simulink model "wetmodel_fixed_angle_r2020"  (R2020b)
settings: Solver=ode45  StartTime=0.0  StopTime=45  RelTol=1e-3  EnableMultiTasking=on
libraries: dspsigops x1
settings Model: Tag=MP_system  Creator=Andries  LastModifiedBy=jurre
settings DataIOCC: LimitDataPoints=on  SaveFormat=Array  SignalLoggingSaveFormat=ModelDataLogs  ReturnWorkspaceOutputs=off
settings OptimizationCC: ExpressionDepthLimit=2147483647  LifeSpan=inf
settings DebuggingCC: UnderspecifiedInitializationDetection=Classic  MergeDetectMultiDrivingBlocksExec=none  SolverPrmCheckMsg=warning  FcnCallInpInsideContextMsg=warning  StateNameClashWarn=warning  SFUnexpectedBacktrackingDiag=warning  SFNoUnconditionalDefaultTransitionDiag=warning  SFExecutionAtInitializationDiag=none  ArithmeticOperatorsInVariantConditions=warning
settings HardwareCC: ProdBitPerPointer=32  ProdBitPerSizeT=32  ProdBitPerPtrDiffT=32  ProdLargestAtomicFloat=None  ProdIntDivRoundTo=Undefined  ProdEndianess=Unspecified  ProdWordSize=32  ProdHWDeviceType=32-bit Generic
settings ModelReferenceCC: PropagateSignalLabelsOutOfModel=off
settings SFSimCC: SimUseLocalCustomCode=off  CustomCodeUndefinedFunction=UseInterfaceOnly
settings RTWCC: RTWUseLocalCustomCode=off
settings CodeAppCC: StateflowObjectComments=on
settings GRTTargetCC: TargetLangStandard=C89/C90 (ANSI)  CombineOutputUpdateFcns=off  GRTInterface=on
settings ConfigComp: CovMetricSettings=dw  CovSaveCumulativeToWorkspaceVar=on  CovSaveSingleToWorkspaceVar=on  CovExternalEMLEnable=off
settings SimscapeCC: SimscapeNormalizeSystem=off

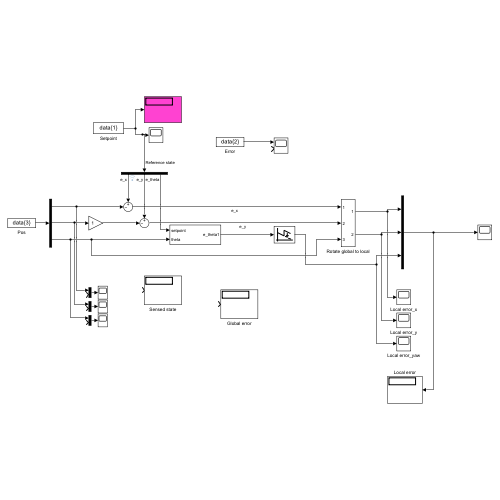
[thumbnail: Simulink's stored preview of the top-level diagram]
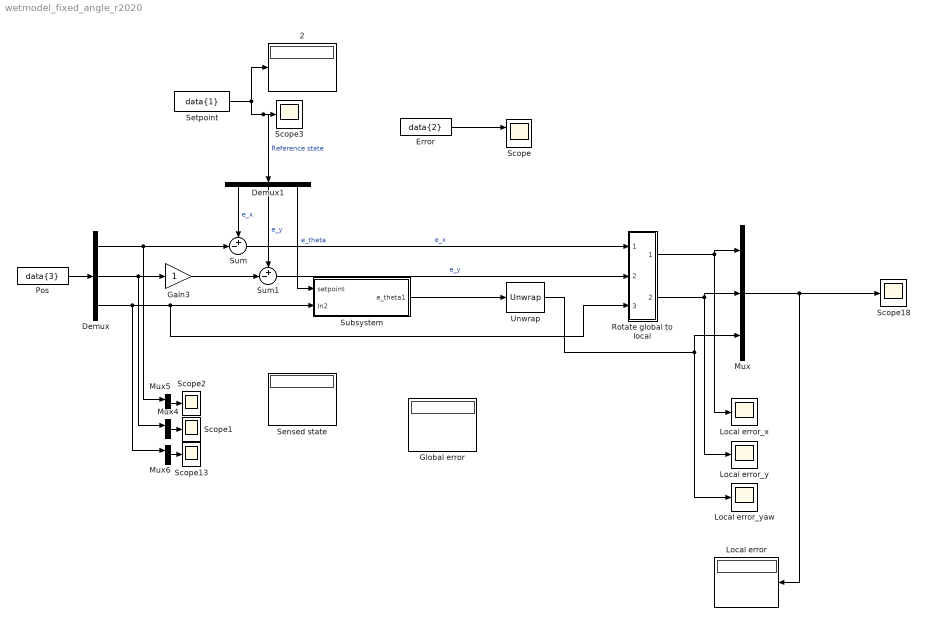
== system wetmodel_fixed_angle_r2020 ==
  "  2" : Display
  Demux : Demux  Outputs=3
  Demux1 : Demux  Outputs=3
  Error : FromWorkspace  VariableName=data{2}
  Gain3 : Gain
  Global error : Display
  Local error : Display
  "Local error_x " : Scope
  "Local error_y " : Scope
  "Local error_yaw " : Scope
  Mux : Mux  Inputs=3
  Mux4 : Mux  Inputs=2
  Mux5 : Mux  Inputs=2
  Mux6 : Mux  Inputs=2
  Pos : FromWorkspace  VariableName=data{3}
  "Rotate global to local " : Subsystem
  Scope : Scope  NumInputPorts=2
  Scope{1..3,13,18} (5 alike) : Scope
  Sensed state : Display
  Setpoint : FromWorkspace  VariableName=data{1}  OutputAfterFinalValue=Holding final value
  Subsystem : Subsystem
  Sum : Sum  Inputs=+-|
  Sum1 : Sum  Inputs=+-|
  Unwrap : dspsigops/Unwrap  tol=pi  InputProcessing=Columns as channels (frame based)  running=off
  wires:
  Setpoint/1 -> "  2"/1, Demux1/1, Scope3/1  "Reference state"
  Sum1/1 -> "Rotate global to local "/2(In2)  "e_y"
  Sum/1 -> "Rotate global to local "/1(In1)  "e_x"
  Mux/1 -> Local error/1, Scope18/1
  "Rotate global to local "/1(Out1) -> Mux/1, "Local error_x "/1
  Demux/1 -> Sum/2, Mux5/1
  Demux/2 -> Mux4/1, Gain3/1
  Demux/3 -> "Rotate global to local "/3(In3), Subsystem/2(In2), Mux6/1
  "Rotate global to local "/2(Out2) -> Mux/2, "Local error_y "/1
  Unwrap/1 -> Mux/3, "Local error_yaw "/1
  Mux6/1 -> Scope13/1
  Mux4/1 -> Scope1/1
  Mux5/1 -> Scope2/1
  Gain3/1 -> Sum1/2
  Pos/1 -> Demux/1
  Error/1 -> Scope/1
  Demux1/1 -> Sum/1  "e_x"
  Demux1/2 -> Sum1/1  "e_y"
  Demux1/3 -> Subsystem/1(setpoint)  "e_theta"
  Subsystem/1(e_theta1) -> Unwrap/1

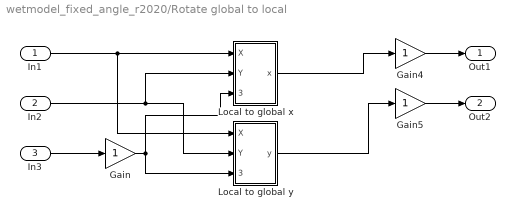
== system wetmodel_fixed_angle_r2020/Rotate global to local  ==
  In1 : Inport
  In2 : Inport  Port=2
  In3 : Inport  Port=3
  Gain : Gain
  Gain4 : Gain
  Gain5 : Gain
  "Local to global x " : Subsystem
  Local to global y : Subsystem
  Out1 : Outport  VectorParamsAs1DForOutWhenUnconnected=off
  Out2 : Outport  Port=2  VectorParamsAs1DForOutWhenUnconnected=off
  wires:
  Local to global y/1(y) -> Gain5/1
  In2/1 -> Local to global y/2(Y), "Local to global x "/2(Y)
  "Local to global x "/1(x) -> Gain4/1
  In1/1 -> Local to global y/1(X), "Local to global x "/1(X)
  In3/1 -> Gain/1
  Gain/1 -> Local to global y/3(theta), "Local to global x "/3(theta)
  Gain5/1 -> Out2/1
  Gain4/1 -> Out1/1

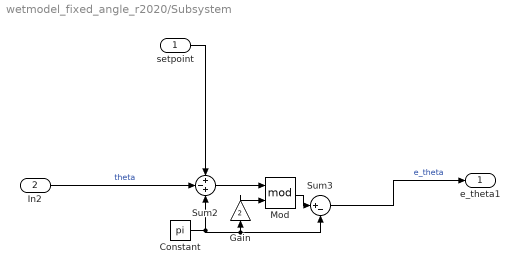
== system wetmodel_fixed_angle_r2020/Subsystem ==
  setpoint : Inport
  In2 : Inport  Port=2
  Constant : Constant  Value=pi
  Gain : Gain  Gain=2
  Mod : Math  Operator=mod  SaturateOnIntegerOverflow=on
  Sum2 : Sum  Inputs=+-+
  Sum3 : Sum  Inputs=|+-
  e_theta1 : Outport
  wires:
  setpoint/1 -> Sum2/1
  Mod/1 -> Sum3/1
  Constant/1 -> Sum3/2, Gain/1, Sum2/3
  In2/1 -> Sum2/2  "theta"
  Gain/1 -> Mod/2
  Sum2/1 -> Mod/1
  Sum3/1 -> e_theta1/1  "e_theta"

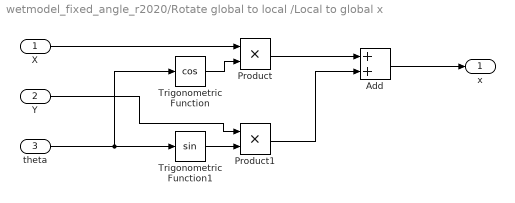
== system wetmodel_fixed_angle_r2020/Rotate global to local /Local to global x  ==
  X : Inport
  Y : Inport  Port=2
  theta : Inport  Port=3
  Add : Sum
  Product : Product
  Product1 : Product
  Trigonometric Function : Trigonometry  Operator=cos
  Trigonometric Function1 : Trigonometry
  x : Outport  VectorParamsAs1DForOutWhenUnconnected=off
  wires:
  Add/1 -> x/1
  Product1/1 -> Add/2
  Product/1 -> Add/1
  Y/1 -> Product1/1
  X/1 -> Product/1
  theta/1 -> Trigonometric Function1/1, Trigonometric Function/1
  Trigonometric Function1/1 -> Product1/2
  Trigonometric Function/1 -> Product/2

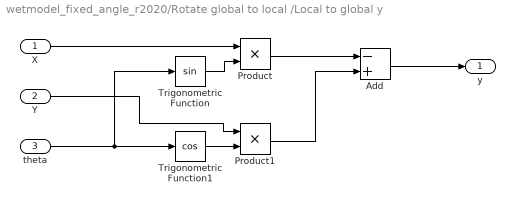
== system wetmodel_fixed_angle_r2020/Rotate global to local /Local to global y ==
  X : Inport
  Y : Inport  Port=2
  theta : Inport  Port=3
  Add : Sum  Inputs=-+
  Product : Product
  Product1 : Product
  Trigonometric Function : Trigonometry
  Trigonometric Function1 : Trigonometry  Operator=cos
  y : Outport  VectorParamsAs1DForOutWhenUnconnected=off
  wires:
  Add/1 -> y/1
  Product1/1 -> Add/2
  Product/1 -> Add/1
  Y/1 -> Product1/1
  X/1 -> Product/1
  theta/1 -> Trigonometric Function1/1, Trigonometric Function/1
  Trigonometric Function1/1 -> Product1/2
  Trigonometric Function/1 -> Product/2
